simulink model "Simulation"  (R2018b)
settings: Solver=VariableStepAuto  StartTime=0.0  StopTime=tmax  RelTol=1e-3
values from neighbouring files (symbols this model uses):
  BPden = [1 alpha]    [RunSimulation.m]
  BPnum = [0.3 alpha]    [RunSimulation.m]
  c = 250    [RunSimulation.m]
  Fb = -1*m    (= -90000)    [RunSimulation.m]
  l = 18    [RunSimulation.m]
  m = 90000    [RunSimulation.m]    (also in TractionCurve.m = 22500)
  p0 = 0    [RunSimulation.m]
  Pres = 0/1000*[5.7/771 0 1.6]    [RunSimulation.m]
  RBD = 5    [RunSimulation.m]
  tl = .1    (= 0.1)    [RunSimulation.m]
  v0 = 100/3.6    (= 27.7777777778)    [RunSimulation.m]
  VBD = 3.5    [RunSimulation.m]
(part 2 of 3)

== system Simulation/Subsystem13/Wagon model2 ==
  p_BP : Inport
  Abs : Abs
  Constant : Constant  Value=m
  Divide : Product  Inputs=*/
  Gain : Gain  Gain=-1/(RBD-VBD)
  Gain1 : Gain  Gain=Fb
  Gravity : Gain  Gain=9.81
  Integrator : Integrator  InitialCondition=v0
  Product : Product
  Rate Limiter : RateLimiter  RisingSlewLimit=1/tf  FallingSlewLimit=-1/tl  SampleTimeMode=inherited
  Saturation : Saturate  UpperLimit=1  LowerLimit=0
  Strahl formula : Polyval  Coefs=Pres
  Sum1 : Sum  Inputs=|+-
  Transfer Fcn : TransferFcn  Numerator=BPnum  Denominator=BPden
  Transport Delay : TransportDelay  DelayTime=l/c  InitialOutput=p0
  Fres : Outport
  p_BP_out : Outport  Port=2
  wires:
  Sum1/1 -> Fres/1, Divide/1  "Fres"
  Strahl formula/1 -> Gravity/1
  Abs/1 -> Strahl formula/1
  Gravity/1 -> Product/2
  Product/1 -> Sum1/2  "Fw"
  Constant/1 -> Product/1, Divide/2
  Divide/1 -> Integrator/1  "a"
  p_BP/1 -> Gain/1, Transport Delay/1
  Gain/1 -> Saturation/1
  Gain1/1 -> Sum1/1
  Saturation/1 -> Rate Limiter/1
  Rate Limiter/1 -> Gain1/1
  Transport Delay/1 -> Transfer Fcn/1
  Transfer Fcn/1 -> p_BP_out/1
  Integrator/1 -> Abs/1  "v"

== system Simulation/Subsystem13/Wagon model3 ==
  p_BP : Inport
  Abs : Abs
  Constant : Constant  Value=m
  Divide : Product  Inputs=*/
  Gain : Gain  Gain=-1/(RBD-VBD)
  Gain1 : Gain  Gain=Fb
  Gravity : Gain  Gain=9.81
  Integrator : Integrator  InitialCondition=v0
  Product : Product
  Rate Limiter : RateLimiter  RisingSlewLimit=1/tf  FallingSlewLimit=-1/tl  SampleTimeMode=inherited
  Saturation : Saturate  UpperLimit=1  LowerLimit=0
  Strahl formula : Polyval  Coefs=Pres
  Sum1 : Sum  Inputs=|+-
  Transfer Fcn : TransferFcn  Numerator=BPnum  Denominator=BPden
  Transport Delay : TransportDelay  DelayTime=l/c  InitialOutput=p0
  Fres : Outport
  p_BP_out : Outport  Port=2
  wires:
  Sum1/1 -> Fres/1, Divide/1  "Fres"
  Strahl formula/1 -> Gravity/1
  Abs/1 -> Strahl formula/1
  Gravity/1 -> Product/2
  Product/1 -> Sum1/2  "Fw"
  Constant/1 -> Product/1, Divide/2
  Divide/1 -> Integrator/1  "a"
  p_BP/1 -> Gain/1, Transport Delay/1
  Gain/1 -> Saturation/1
  Gain1/1 -> Sum1/1
  Saturation/1 -> Rate Limiter/1
  Rate Limiter/1 -> Gain1/1
  Transport Delay/1 -> Transfer Fcn/1
  Transfer Fcn/1 -> p_BP_out/1
  Integrator/1 -> Abs/1  "v"

== system Simulation/Subsystem13/Wagon model4 ==
  p_BP : Inport
  Abs : Abs
  Constant : Constant  Value=m
  Divide : Product  Inputs=*/
  Gain : Gain  Gain=-1/(RBD-VBD)
  Gain1 : Gain  Gain=Fb
  Gravity : Gain  Gain=9.81
  Integrator : Integrator  InitialCondition=v0
  Product : Product
  Rate Limiter : RateLimiter  RisingSlewLimit=1/tf  FallingSlewLimit=-1/tl  SampleTimeMode=inherited
  Saturation : Saturate  UpperLimit=1  LowerLimit=0
  Strahl formula : Polyval  Coefs=Pres
  Sum1 : Sum  Inputs=|+-
  Transfer Fcn : TransferFcn  Numerator=BPnum  Denominator=BPden
  Transport Delay : TransportDelay  DelayTime=l/c  InitialOutput=p0
  Fres : Outport
  p_BP_out : Outport  Port=2
  wires:
  Sum1/1 -> Fres/1, Divide/1  "Fres"
  Strahl formula/1 -> Gravity/1
  Abs/1 -> Strahl formula/1
  Gravity/1 -> Product/2
  Product/1 -> Sum1/2  "Fw"
  Integrator/1 -> Abs/1  "v"
  Constant/1 -> Product/1, Divide/2
  Divide/1 -> Integrator/1  "a"
  p_BP/1 -> Gain/1, Transport Delay/1
  Gain/1 -> Saturation/1
  Gain1/1 -> Sum1/1
  Saturation/1 -> Rate Limiter/1
  Rate Limiter/1 -> Gain1/1
  Transfer Fcn/1 -> p_BP_out/1
  Transport Delay/1 -> Transfer Fcn/1

== system Simulation/Subsystem14/Wagon model ==
  p_BP : Inport
  Abs : Abs
  Constant : Constant  Value=m
  Divide : Product  Inputs=*/
  Gain : Gain  Gain=-1/(RBD-VBD)
  Gain1 : Gain  Gain=Fb
  Gravity : Gain  Gain=9.81
  Integrator : Integrator  InitialCondition=v0
  Product : Product
  Rate Limiter : RateLimiter  RisingSlewLimit=1/tf  FallingSlewLimit=-1/tl  SampleTimeMode=inherited
  Saturation : Saturate  UpperLimit=1  LowerLimit=0
  Strahl formula : Polyval  Coefs=Pres
  Sum1 : Sum  Inputs=|+-
  Transfer Fcn : TransferFcn  Numerator=BPnum  Denominator=BPden
  Transport Delay : TransportDelay  DelayTime=l/c  InitialOutput=p0
  Fres : Outport
  p_BP_out : Outport  Port=2
  wires:
  Sum1/1 -> Fres/1, Divide/1  "Fres"
  Strahl formula/1 -> Gravity/1
  Abs/1 -> Strahl formula/1
  Gravity/1 -> Product/2
  Product/1 -> Sum1/2  "Fw"
  Integrator/1 -> Abs/1  "v"
  Constant/1 -> Product/1, Divide/2
  Divide/1 -> Integrator/1  "a"
  p_BP/1 -> Gain/1, Transport Delay/1
  Gain/1 -> Saturation/1
  Gain1/1 -> Sum1/1
  Saturation/1 -> Rate Limiter/1
  Rate Limiter/1 -> Gain1/1
  Transfer Fcn/1 -> p_BP_out/1
  Transport Delay/1 -> Transfer Fcn/1

== system Simulation/Subsystem14/Wagon model1 ==
  p_BP : Inport
  Abs : Abs
  Constant : Constant  Value=m
  Divide : Product  Inputs=*/
  Gain : Gain  Gain=-1/(RBD-VBD)
  Gain1 : Gain  Gain=Fb
  Gravity : Gain  Gain=9.81
  Integrator : Integrator  InitialCondition=v0
  Product : Product
  Rate Limiter : RateLimiter  RisingSlewLimit=1/tf  FallingSlewLimit=-1/tl  SampleTimeMode=inherited
  Saturation : Saturate  UpperLimit=1  LowerLimit=0
  Strahl formula : Polyval  Coefs=Pres
  Sum1 : Sum  Inputs=|+-
  Transfer Fcn : TransferFcn  Numerator=BPnum  Denominator=BPden
  Transport Delay : TransportDelay  DelayTime=l/c  InitialOutput=p0
  Fres : Outport
  p_BP_out : Outport  Port=2
  wires:
  Sum1/1 -> Fres/1, Divide/1  "Fres"
  Strahl formula/1 -> Gravity/1
  Abs/1 -> Strahl formula/1
  Gravity/1 -> Product/2
  Product/1 -> Sum1/2  "Fw"
  Integrator/1 -> Abs/1  "v"
  Constant/1 -> Product/1, Divide/2
  Divide/1 -> Integrator/1  "a"
  p_BP/1 -> Gain/1, Transport Delay/1
  Gain/1 -> Saturation/1
  Gain1/1 -> Sum1/1
  Saturation/1 -> Rate Limiter/1
  Rate Limiter/1 -> Gain1/1
  Transport Delay/1 -> Transfer Fcn/1
  Transfer Fcn/1 -> p_BP_out/1

== system Simulation/Subsystem14/Wagon model2 ==
  p_BP : Inport
  Abs : Abs
  Constant : Constant  Value=m
  Divide : Product  Inputs=*/
  Gain : Gain  Gain=-1/(RBD-VBD)
  Gain1 : Gain  Gain=Fb
  Gravity : Gain  Gain=9.81
  Integrator : Integrator  InitialCondition=v0
  Product : Product
  Rate Limiter : RateLimiter  RisingSlewLimit=1/tf  FallingSlewLimit=-1/tl  SampleTimeMode=inherited
  Saturation : Saturate  UpperLimit=1  LowerLimit=0
  Strahl formula : Polyval  Coefs=Pres
  Sum1 : Sum  Inputs=|+-
  Transfer Fcn : TransferFcn  Numerator=BPnum  Denominator=BPden
  Transport Delay : TransportDelay  DelayTime=l/c  InitialOutput=p0
  Fres : Outport
  p_BP_out : Outport  Port=2
  wires:
  Sum1/1 -> Fres/1, Divide/1  "Fres"
  Strahl formula/1 -> Gravity/1
  Abs/1 -> Strahl formula/1
  Gravity/1 -> Product/2
  Product/1 -> Sum1/2  "Fw"
  Constant/1 -> Product/1, Divide/2
  Divide/1 -> Integrator/1  "a"
  p_BP/1 -> Gain/1, Transport Delay/1
  Gain/1 -> Saturation/1
  Gain1/1 -> Sum1/1
  Saturation/1 -> Rate Limiter/1
  Rate Limiter/1 -> Gain1/1
  Transport Delay/1 -> Transfer Fcn/1
  Transfer Fcn/1 -> p_BP_out/1
  Integrator/1 -> Abs/1  "v"

== system Simulation/Subsystem14/Wagon model3 ==
  p_BP : Inport
  Abs : Abs
  Constant : Constant  Value=m
  Divide : Product  Inputs=*/
  Gain : Gain  Gain=-1/(RBD-VBD)
  Gain1 : Gain  Gain=Fb
  Gravity : Gain  Gain=9.81
  Integrator : Integrator  InitialCondition=v0
  Product : Product
  Rate Limiter : RateLimiter  RisingSlewLimit=1/tf  FallingSlewLimit=-1/tl  SampleTimeMode=inherited
  Saturation : Saturate  UpperLimit=1  LowerLimit=0
  Strahl formula : Polyval  Coefs=Pres
  Sum1 : Sum  Inputs=|+-
  Transfer Fcn : TransferFcn  Numerator=BPnum  Denominator=BPden
  Transport Delay : TransportDelay  DelayTime=l/c  InitialOutput=p0
  Fres : Outport
  p_BP_out : Outport  Port=2
  wires:
  Sum1/1 -> Fres/1, Divide/1  "Fres"
  Strahl formula/1 -> Gravity/1
  Abs/1 -> Strahl formula/1
  Gravity/1 -> Product/2
  Product/1 -> Sum1/2  "Fw"
  Constant/1 -> Product/1, Divide/2
  Divide/1 -> Integrator/1  "a"
  p_BP/1 -> Gain/1, Transport Delay/1
  Gain/1 -> Saturation/1
  Gain1/1 -> Sum1/1
  Saturation/1 -> Rate Limiter/1
  Rate Limiter/1 -> Gain1/1
  Transport Delay/1 -> Transfer Fcn/1
  Transfer Fcn/1 -> p_BP_out/1
  Integrator/1 -> Abs/1  "v"

== system Simulation/Subsystem14/Wagon model4 ==
  p_BP : Inport
  Abs : Abs
  Constant : Constant  Value=m
  Divide : Product  Inputs=*/
  Gain : Gain  Gain=-1/(RBD-VBD)
  Gain1 : Gain  Gain=Fb
  Gravity : Gain  Gain=9.81
  Integrator : Integrator  InitialCondition=v0
  Product : Product
  Rate Limiter : RateLimiter  RisingSlewLimit=1/tf  FallingSlewLimit=-1/tl  SampleTimeMode=inherited
  Saturation : Saturate  UpperLimit=1  LowerLimit=0
  Strahl formula : Polyval  Coefs=Pres
  Sum1 : Sum  Inputs=|+-
  Transfer Fcn : TransferFcn  Numerator=BPnum  Denominator=BPden
  Transport Delay : TransportDelay  DelayTime=l/c  InitialOutput=p0
  Fres : Outport
  p_BP_out : Outport  Port=2
  wires:
  Sum1/1 -> Fres/1, Divide/1  "Fres"
  Strahl formula/1 -> Gravity/1
  Abs/1 -> Strahl formula/1
  Gravity/1 -> Product/2
  Product/1 -> Sum1/2  "Fw"
  Integrator/1 -> Abs/1  "v"
  Constant/1 -> Product/1, Divide/2
  Divide/1 -> Integrator/1  "a"
  p_BP/1 -> Gain/1, Transport Delay/1
  Gain/1 -> Saturation/1
  Gain1/1 -> Sum1/1
  Saturation/1 -> Rate Limiter/1
  Rate Limiter/1 -> Gain1/1
  Transfer Fcn/1 -> p_BP_out/1
  Transport Delay/1 -> Transfer Fcn/1

== system Simulation/Subsystem15/Wagon model ==
  p_BP : Inport
  Abs : Abs
  Constant : Constant  Value=m
  Divide : Product  Inputs=*/
  Gain : Gain  Gain=-1/(RBD-VBD)
  Gain1 : Gain  Gain=Fb
  Gravity : Gain  Gain=9.81
  Integrator : Integrator  InitialCondition=v0
  Product : Product
  Rate Limiter : RateLimiter  RisingSlewLimit=1/tf  FallingSlewLimit=-1/tl  SampleTimeMode=inherited
  Saturation : Saturate  UpperLimit=1  LowerLimit=0
  Strahl formula : Polyval  Coefs=Pres
  Sum1 : Sum  Inputs=|+-
  Transfer Fcn : TransferFcn  Numerator=BPnum  Denominator=BPden
  Transport Delay : TransportDelay  DelayTime=l/c  InitialOutput=p0
  Fres : Outport
  p_BP_out : Outport  Port=2
  wires:
  Sum1/1 -> Fres/1, Divide/1  "Fres"
  Strahl formula/1 -> Gravity/1
  Abs/1 -> Strahl formula/1
  Gravity/1 -> Product/2
  Product/1 -> Sum1/2  "Fw"
  Integrator/1 -> Abs/1  "v"
  Constant/1 -> Product/1, Divide/2
  Divide/1 -> Integrator/1  "a"
  p_BP/1 -> Gain/1, Transport Delay/1
  Gain/1 -> Saturation/1
  Gain1/1 -> Sum1/1
  Saturation/1 -> Rate Limiter/1
  Rate Limiter/1 -> Gain1/1
  Transfer Fcn/1 -> p_BP_out/1
  Transport Delay/1 -> Transfer Fcn/1

== system Simulation/Subsystem15/Wagon model1 ==
  p_BP : Inport
  Abs : Abs
  Constant : Constant  Value=m
  Divide : Product  Inputs=*/
  Gain : Gain  Gain=-1/(RBD-VBD)
  Gain1 : Gain  Gain=Fb
  Gravity : Gain  Gain=9.81
  Integrator : Integrator  InitialCondition=v0
  Product : Product
  Rate Limiter : RateLimiter  RisingSlewLimit=1/tf  FallingSlewLimit=-1/tl  SampleTimeMode=inherited
  Saturation : Saturate  UpperLimit=1  LowerLimit=0
  Strahl formula : Polyval  Coefs=Pres
  Sum1 : Sum  Inputs=|+-
  Transfer Fcn : TransferFcn  Numerator=BPnum  Denominator=BPden
  Transport Delay : TransportDelay  DelayTime=l/c  InitialOutput=p0
  Fres : Outport
  p_BP_out : Outport  Port=2
  wires:
  Sum1/1 -> Fres/1, Divide/1  "Fres"
  Strahl formula/1 -> Gravity/1
  Abs/1 -> Strahl formula/1
  Gravity/1 -> Product/2
  Product/1 -> Sum1/2  "Fw"
  Integrator/1 -> Abs/1  "v"
  Constant/1 -> Product/1, Divide/2
  Divide/1 -> Integrator/1  "a"
  p_BP/1 -> Gain/1, Transport Delay/1
  Gain/1 -> Saturation/1
  Gain1/1 -> Sum1/1
  Saturation/1 -> Rate Limiter/1
  Rate Limiter/1 -> Gain1/1
  Transport Delay/1 -> Transfer Fcn/1
  Transfer Fcn/1 -> p_BP_out/1

== system Simulation/Subsystem15/Wagon model2 ==
  p_BP : Inport
  Abs : Abs
  Constant : Constant  Value=m
  Divide : Product  Inputs=*/
  Gain : Gain  Gain=-1/(RBD-VBD)
  Gain1 : Gain  Gain=Fb
  Gravity : Gain  Gain=9.81
  Integrator : Integrator  InitialCondition=v0
  Product : Product
  Rate Limiter : RateLimiter  RisingSlewLimit=1/tf  FallingSlewLimit=-1/tl  SampleTimeMode=inherited
  Saturation : Saturate  UpperLimit=1  LowerLimit=0
  Strahl formula : Polyval  Coefs=Pres
  Sum1 : Sum  Inputs=|+-
  Transfer Fcn : TransferFcn  Numerator=BPnum  Denominator=BPden
  Transport Delay : TransportDelay  DelayTime=l/c  InitialOutput=p0
  Fres : Outport
  p_BP_out : Outport  Port=2
  wires:
  Sum1/1 -> Fres/1, Divide/1  "Fres"
  Strahl formula/1 -> Gravity/1
  Abs/1 -> Strahl formula/1
  Gravity/1 -> Product/2
  Product/1 -> Sum1/2  "Fw"
  Constant/1 -> Product/1, Divide/2
  Divide/1 -> Integrator/1  "a"
  p_BP/1 -> Gain/1, Transport Delay/1
  Gain/1 -> Saturation/1
  Gain1/1 -> Sum1/1
  Saturation/1 -> Rate Limiter/1
  Rate Limiter/1 -> Gain1/1
  Transport Delay/1 -> Transfer Fcn/1
  Transfer Fcn/1 -> p_BP_out/1
  Integrator/1 -> Abs/1  "v"

== system Simulation/Subsystem15/Wagon model3 ==
  p_BP : Inport
  Abs : Abs
  Constant : Constant  Value=m
  Divide : Product  Inputs=*/
  Gain : Gain  Gain=-1/(RBD-VBD)
  Gain1 : Gain  Gain=Fb
  Gravity : Gain  Gain=9.81
  Integrator : Integrator  InitialCondition=v0
  Product : Product
  Rate Limiter : RateLimiter  RisingSlewLimit=1/tf  FallingSlewLimit=-1/tl  SampleTimeMode=inherited
  Saturation : Saturate  UpperLimit=1  LowerLimit=0
  Strahl formula : Polyval  Coefs=Pres
  Sum1 : Sum  Inputs=|+-
  Transfer Fcn : TransferFcn  Numerator=BPnum  Denominator=BPden
  Transport Delay : TransportDelay  DelayTime=l/c  InitialOutput=p0
  Fres : Outport
  p_BP_out : Outport  Port=2
  wires:
  Sum1/1 -> Fres/1, Divide/1  "Fres"
  Strahl formula/1 -> Gravity/1
  Abs/1 -> Strahl formula/1
  Gravity/1 -> Product/2
  Product/1 -> Sum1/2  "Fw"
  Integrator/1 -> Abs/1  "v"
  Constant/1 -> Product/1, Divide/2
  Divide/1 -> Integrator/1  "a"
  p_BP/1 -> Gain/1, Transport Delay/1
  Gain/1 -> Saturation/1
  Gain1/1 -> Sum1/1
  Saturation/1 -> Rate Limiter/1
  Rate Limiter/1 -> Gain1/1
  Transport Delay/1 -> Transfer Fcn/1
  Transfer Fcn/1 -> p_BP_out/1

== system Simulation/Subsystem15/Wagon model4 ==
  p_BP : Inport
  Abs : Abs
  Constant : Constant  Value=m
  Divide : Product  Inputs=*/
  Gain : Gain  Gain=-1/(RBD-VBD)
  Gain1 : Gain  Gain=Fb
  Gravity : Gain  Gain=9.81
  Integrator : Integrator  InitialCondition=v0
  Product : Product
  Rate Limiter : RateLimiter  RisingSlewLimit=1/tf  FallingSlewLimit=-1/tl  SampleTimeMode=inherited
  Saturation : Saturate  UpperLimit=1  LowerLimit=0
  Strahl formula : Polyval  Coefs=Pres
  Sum1 : Sum  Inputs=|+-
  Transfer Fcn : TransferFcn  Numerator=BPnum  Denominator=BPden
  Transport Delay : TransportDelay  DelayTime=l/c  InitialOutput=p0
  Fres : Outport
  p_BP_out : Outport  Port=2
  wires:
  Sum1/1 -> Fres/1, Divide/1  "Fres"
  Strahl formula/1 -> Gravity/1
  Abs/1 -> Strahl formula/1
  Gravity/1 -> Product/2
  Product/1 -> Sum1/2  "Fw"
  Integrator/1 -> Abs/1  "v"
  Constant/1 -> Product/1, Divide/2
  Divide/1 -> Integrator/1  "a"
  p_BP/1 -> Gain/1, Transport Delay/1
  Gain/1 -> Saturation/1
  Gain1/1 -> Sum1/1
  Saturation/1 -> Rate Limiter/1
  Rate Limiter/1 -> Gain1/1
  Transfer Fcn/1 -> p_BP_out/1
  Transport Delay/1 -> Transfer Fcn/1

== system Simulation/Subsystem2/Wagon model ==
  p_BP : Inport
  Abs : Abs
  Constant : Constant  Value=m
  Divide : Product  Inputs=*/
  Gain : Gain  Gain=-1/(RBD-VBD)
  Gain1 : Gain  Gain=Fb
  Gravity : Gain  Gain=9.81
  Integrator : Integrator  InitialCondition=v0
  Product : Product
  Rate Limiter : RateLimiter  RisingSlewLimit=1/tf  FallingSlewLimit=-1/tl  SampleTimeMode=inherited
  Saturation : Saturate  UpperLimit=1  LowerLimit=0
  Strahl formula : Polyval  Coefs=Pres
  Sum1 : Sum  Inputs=|+-
  Transfer Fcn : TransferFcn  Numerator=BPnum  Denominator=BPden
  Transport Delay : TransportDelay  DelayTime=l/c  InitialOutput=p0
  Fres : Outport
  p_BP_out : Outport  Port=2
  wires:
  Sum1/1 -> Fres/1, Divide/1  "Fres"
  Strahl formula/1 -> Gravity/1
  Abs/1 -> Strahl formula/1
  Gravity/1 -> Product/2
  Product/1 -> Sum1/2  "Fw"
  Integrator/1 -> Abs/1  "v"
  Constant/1 -> Product/1, Divide/2
  Divide/1 -> Integrator/1  "a"
  p_BP/1 -> Gain/1, Transport Delay/1
  Gain/1 -> Saturation/1
  Gain1/1 -> Sum1/1
  Saturation/1 -> Rate Limiter/1
  Rate Limiter/1 -> Gain1/1
  Transfer Fcn/1 -> p_BP_out/1
  Transport Delay/1 -> Transfer Fcn/1

== system Simulation/Subsystem2/Wagon model1 ==
  p_BP : Inport
  Abs : Abs
  Constant : Constant  Value=m
  Divide : Product  Inputs=*/
  Gain : Gain  Gain=-1/(RBD-VBD)
  Gain1 : Gain  Gain=Fb
  Gravity : Gain  Gain=9.81
  Integrator : Integrator  InitialCondition=v0
  Product : Product
  Rate Limiter : RateLimiter  RisingSlewLimit=1/tf  FallingSlewLimit=-1/tl  SampleTimeMode=inherited
  Saturation : Saturate  UpperLimit=1  LowerLimit=0
  Strahl formula : Polyval  Coefs=Pres
  Sum1 : Sum  Inputs=|+-
  Transfer Fcn : TransferFcn  Numerator=BPnum  Denominator=BPden
  Transport Delay : TransportDelay  DelayTime=l/c  InitialOutput=p0
  Fres : Outport
  p_BP_out : Outport  Port=2
  wires:
  Sum1/1 -> Fres/1, Divide/1  "Fres"
  Strahl formula/1 -> Gravity/1
  Abs/1 -> Strahl formula/1
  Gravity/1 -> Product/2
  Product/1 -> Sum1/2  "Fw"
  Integrator/1 -> Abs/1  "v"
  Constant/1 -> Product/1, Divide/2
  Divide/1 -> Integrator/1  "a"
  p_BP/1 -> Gain/1, Transport Delay/1
  Gain/1 -> Saturation/1
  Gain1/1 -> Sum1/1
  Saturation/1 -> Rate Limiter/1
  Rate Limiter/1 -> Gain1/1
  Transport Delay/1 -> Transfer Fcn/1
  Transfer Fcn/1 -> p_BP_out/1

== system Simulation/Subsystem2/Wagon model2 ==
  p_BP : Inport
  Abs : Abs
  Constant : Constant  Value=m
  Divide : Product  Inputs=*/
  Gain : Gain  Gain=-1/(RBD-VBD)
  Gain1 : Gain  Gain=Fb
  Gravity : Gain  Gain=9.81
  Integrator : Integrator  InitialCondition=v0
  Product : Product
  Rate Limiter : RateLimiter  RisingSlewLimit=1/tf  FallingSlewLimit=-1/tl  SampleTimeMode=inherited
  Saturation : Saturate  UpperLimit=1  LowerLimit=0
  Strahl formula : Polyval  Coefs=Pres
  Sum1 : Sum  Inputs=|+-
  Transfer Fcn : TransferFcn  Numerator=BPnum  Denominator=BPden
  Transport Delay : TransportDelay  DelayTime=l/c  InitialOutput=p0
  Fres : Outport
  p_BP_out : Outport  Port=2
  wires:
  Sum1/1 -> Fres/1, Divide/1  "Fres"
  Strahl formula/1 -> Gravity/1
  Abs/1 -> Strahl formula/1
  Gravity/1 -> Product/2
  Product/1 -> Sum1/2  "Fw"
  Constant/1 -> Product/1, Divide/2
  Divide/1 -> Integrator/1  "a"
  p_BP/1 -> Gain/1, Transport Delay/1
  Gain/1 -> Saturation/1
  Gain1/1 -> Sum1/1
  Saturation/1 -> Rate Limiter/1
  Rate Limiter/1 -> Gain1/1
  Transport Delay/1 -> Transfer Fcn/1
  Transfer Fcn/1 -> p_BP_out/1
  Integrator/1 -> Abs/1  "v"

== system Simulation/Subsystem2/Wagon model3 ==
  p_BP : Inport
  Abs : Abs
  Constant : Constant  Value=m
  Divide : Product  Inputs=*/
  Gain : Gain  Gain=-1/(RBD-VBD)
  Gain1 : Gain  Gain=Fb
  Gravity : Gain  Gain=9.81
  Integrator : Integrator  InitialCondition=v0
  Product : Product
  Rate Limiter : RateLimiter  RisingSlewLimit=1/tf  FallingSlewLimit=-1/tl  SampleTimeMode=inherited
  Saturation : Saturate  UpperLimit=1  LowerLimit=0
  Strahl formula : Polyval  Coefs=Pres
  Sum1 : Sum  Inputs=|+-
  Transfer Fcn : TransferFcn  Numerator=BPnum  Denominator=BPden
  Transport Delay : TransportDelay  DelayTime=l/c  InitialOutput=p0
  Fres : Outport
  p_BP_out : Outport  Port=2
  wires:
  Sum1/1 -> Fres/1, Divide/1  "Fres"
  Strahl formula/1 -> Gravity/1
  Abs/1 -> Strahl formula/1
  Gravity/1 -> Product/2
  Product/1 -> Sum1/2  "Fw"
  Constant/1 -> Product/1, Divide/2
  Divide/1 -> Integrator/1  "a"
  p_BP/1 -> Gain/1, Transport Delay/1
  Gain/1 -> Saturation/1
  Gain1/1 -> Sum1/1
  Saturation/1 -> Rate Limiter/1
  Rate Limiter/1 -> Gain1/1
  Transport Delay/1 -> Transfer Fcn/1
  Transfer Fcn/1 -> p_BP_out/1
  Integrator/1 -> Abs/1  "v"

== system Simulation/Subsystem2/Wagon model4 ==
  p_BP : Inport
  Abs : Abs
  Constant : Constant  Value=m
  Divide : Product  Inputs=*/
  Gain : Gain  Gain=-1/(RBD-VBD)
  Gain1 : Gain  Gain=Fb
  Gravity : Gain  Gain=9.81
  Integrator : Integrator  InitialCondition=v0
  Product : Product
  Rate Limiter : RateLimiter  RisingSlewLimit=1/tf  FallingSlewLimit=-1/tl  SampleTimeMode=inherited
  Saturation : Saturate  UpperLimit=1  LowerLimit=0
  Strahl formula : Polyval  Coefs=Pres
  Sum1 : Sum  Inputs=|+-
  Transfer Fcn : TransferFcn  Numerator=BPnum  Denominator=BPden
  Transport Delay : TransportDelay  DelayTime=l/c  InitialOutput=p0
  Fres : Outport
  p_BP_out : Outport  Port=2
  wires:
  Sum1/1 -> Fres/1, Divide/1  "Fres"
  Strahl formula/1 -> Gravity/1
  Abs/1 -> Strahl formula/1
  Gravity/1 -> Product/2
  Product/1 -> Sum1/2  "Fw"
  Integrator/1 -> Abs/1  "v"
  Constant/1 -> Product/1, Divide/2
  Divide/1 -> Integrator/1  "a"
  p_BP/1 -> Gain/1, Transport Delay/1
  Gain/1 -> Saturation/1
  Gain1/1 -> Sum1/1
  Saturation/1 -> Rate Limiter/1
  Rate Limiter/1 -> Gain1/1
  Transfer Fcn/1 -> p_BP_out/1
  Transport Delay/1 -> Transfer Fcn/1

== system Simulation/Subsystem3/Wagon model ==
  p_BP : Inport
  Abs : Abs
  Constant : Constant  Value=m
  Divide : Product  Inputs=*/
  Gain : Gain  Gain=-1/(RBD-VBD)
  Gain1 : Gain  Gain=Fb
  Gravity : Gain  Gain=9.81
  Integrator : Integrator  InitialCondition=v0
  Product : Product
  Rate Limiter : RateLimiter  RisingSlewLimit=1/tf  FallingSlewLimit=-1/tl  SampleTimeMode=inherited
  Saturation : Saturate  UpperLimit=1  LowerLimit=0
  Strahl formula : Polyval  Coefs=Pres
  Sum1 : Sum  Inputs=|+-
  Transfer Fcn : TransferFcn  Numerator=BPnum  Denominator=BPden
  Transport Delay : TransportDelay  DelayTime=l/c  InitialOutput=p0
  Fres : Outport
  p_BP_out : Outport  Port=2
  wires:
  Sum1/1 -> Fres/1, Divide/1  "Fres"
  Strahl formula/1 -> Gravity/1
  Abs/1 -> Strahl formula/1
  Gravity/1 -> Product/2
  Product/1 -> Sum1/2  "Fw"
  Integrator/1 -> Abs/1  "v"
  Constant/1 -> Product/1, Divide/2
  Divide/1 -> Integrator/1  "a"
  p_BP/1 -> Gain/1, Transport Delay/1
  Gain/1 -> Saturation/1
  Gain1/1 -> Sum1/1
  Saturation/1 -> Rate Limiter/1
  Rate Limiter/1 -> Gain1/1
  Transfer Fcn/1 -> p_BP_out/1
  Transport Delay/1 -> Transfer Fcn/1

== system Simulation/Subsystem3/Wagon model1 ==
  p_BP : Inport
  Abs : Abs
  Constant : Constant  Value=m
  Divide : Product  Inputs=*/
  Gain : Gain  Gain=-1/(RBD-VBD)
  Gain1 : Gain  Gain=Fb
  Gravity : Gain  Gain=9.81
  Integrator : Integrator  InitialCondition=v0
  Product : Product
  Rate Limiter : RateLimiter  RisingSlewLimit=1/tf  FallingSlewLimit=-1/tl  SampleTimeMode=inherited
  Saturation : Saturate  UpperLimit=1  LowerLimit=0
  Strahl formula : Polyval  Coefs=Pres
  Sum1 : Sum  Inputs=|+-
  Transfer Fcn : TransferFcn  Numerator=BPnum  Denominator=BPden
  Transport Delay : TransportDelay  DelayTime=l/c  InitialOutput=p0
  Fres : Outport
  p_BP_out : Outport  Port=2
  wires:
  Sum1/1 -> Fres/1, Divide/1  "Fres"
  Strahl formula/1 -> Gravity/1
  Abs/1 -> Strahl formula/1
  Gravity/1 -> Product/2
  Product/1 -> Sum1/2  "Fw"
  Integrator/1 -> Abs/1  "v"
  Constant/1 -> Product/1, Divide/2
  Divide/1 -> Integrator/1  "a"
  p_BP/1 -> Gain/1, Transport Delay/1
  Gain/1 -> Saturation/1
  Gain1/1 -> Sum1/1
  Saturation/1 -> Rate Limiter/1
  Rate Limiter/1 -> Gain1/1
  Transport Delay/1 -> Transfer Fcn/1
  Transfer Fcn/1 -> p_BP_out/1

== system Simulation/Subsystem3/Wagon model2 ==
  p_BP : Inport
  Abs : Abs
  Constant : Constant  Value=m
  Divide : Product  Inputs=*/
  Gain : Gain  Gain=-1/(RBD-VBD)
  Gain1 : Gain  Gain=Fb
  Gravity : Gain  Gain=9.81
  Integrator : Integrator  InitialCondition=v0
  Product : Product
  Rate Limiter : RateLimiter  RisingSlewLimit=1/tf  FallingSlewLimit=-1/tl  SampleTimeMode=inherited
  Saturation : Saturate  UpperLimit=1  LowerLimit=0
  Strahl formula : Polyval  Coefs=Pres
  Sum1 : Sum  Inputs=|+-
  Transfer Fcn : TransferFcn  Numerator=BPnum  Denominator=BPden
  Transport Delay : TransportDelay  DelayTime=l/c  InitialOutput=p0
  Fres : Outport
  p_BP_out : Outport  Port=2
  wires:
  Sum1/1 -> Fres/1, Divide/1  "Fres"
  Strahl formula/1 -> Gravity/1
  Abs/1 -> Strahl formula/1
  Gravity/1 -> Product/2
  Product/1 -> Sum1/2  "Fw"
  Constant/1 -> Product/1, Divide/2
  Divide/1 -> Integrator/1  "a"
  p_BP/1 -> Gain/1, Transport Delay/1
  Gain/1 -> Saturation/1
  Gain1/1 -> Sum1/1
  Saturation/1 -> Rate Limiter/1
  Rate Limiter/1 -> Gain1/1
  Transport Delay/1 -> Transfer Fcn/1
  Transfer Fcn/1 -> p_BP_out/1
  Integrator/1 -> Abs/1  "v"

== system Simulation/Subsystem3/Wagon model3 ==
  p_BP : Inport
  Abs : Abs
  Constant : Constant  Value=m
  Divide : Product  Inputs=*/
  Gain : Gain  Gain=-1/(RBD-VBD)
  Gain1 : Gain  Gain=Fb
  Gravity : Gain  Gain=9.81
  Integrator : Integrator  InitialCondition=v0
  Product : Product
  Rate Limiter : RateLimiter  RisingSlewLimit=1/tf  FallingSlewLimit=-1/tl  SampleTimeMode=inherited
  Saturation : Saturate  UpperLimit=1  LowerLimit=0
  Strahl formula : Polyval  Coefs=Pres
  Sum1 : Sum  Inputs=|+-
  Transfer Fcn : TransferFcn  Numerator=BPnum  Denominator=BPden
  Transport Delay : TransportDelay  DelayTime=l/c  InitialOutput=p0
  Fres : Outport
  p_BP_out : Outport  Port=2
  wires:
  Sum1/1 -> Fres/1, Divide/1  "Fres"
  Strahl formula/1 -> Gravity/1
  Abs/1 -> Strahl formula/1
  Gravity/1 -> Product/2
  Product/1 -> Sum1/2  "Fw"
  Constant/1 -> Product/1, Divide/2
  Divide/1 -> Integrator/1  "a"
  p_BP/1 -> Gain/1, Transport Delay/1
  Gain/1 -> Saturation/1
  Gain1/1 -> Sum1/1
  Saturation/1 -> Rate Limiter/1
  Rate Limiter/1 -> Gain1/1
  Transport Delay/1 -> Transfer Fcn/1
  Transfer Fcn/1 -> p_BP_out/1
  Integrator/1 -> Abs/1  "v"

== system Simulation/Subsystem3/Wagon model4 ==
  p_BP : Inport
  Abs : Abs
  Constant : Constant  Value=m
  Divide : Product  Inputs=*/
  Gain : Gain  Gain=-1/(RBD-VBD)
  Gain1 : Gain  Gain=Fb
  Gravity : Gain  Gain=9.81
  Integrator : Integrator  InitialCondition=v0
  Product : Product
  Rate Limiter : RateLimiter  RisingSlewLimit=1/tf  FallingSlewLimit=-1/tl  SampleTimeMode=inherited
  Saturation : Saturate  UpperLimit=1  LowerLimit=0
  Strahl formula : Polyval  Coefs=Pres
  Sum1 : Sum  Inputs=|+-
  Transfer Fcn : TransferFcn  Numerator=BPnum  Denominator=BPden
  Transport Delay : TransportDelay  DelayTime=l/c  InitialOutput=p0
  Fres : Outport
  p_BP_out : Outport  Port=2
  wires:
  Sum1/1 -> Fres/1, Divide/1  "Fres"
  Strahl formula/1 -> Gravity/1
  Abs/1 -> Strahl formula/1
  Gravity/1 -> Product/2
  Product/1 -> Sum1/2  "Fw"
  Integrator/1 -> Abs/1  "v"
  Constant/1 -> Product/1, Divide/2
  Divide/1 -> Integrator/1  "a"
  p_BP/1 -> Gain/1, Transport Delay/1
  Gain/1 -> Saturation/1
  Gain1/1 -> Sum1/1
  Saturation/1 -> Rate Limiter/1
  Rate Limiter/1 -> Gain1/1
  Transfer Fcn/1 -> p_BP_out/1
  Transport Delay/1 -> Transfer Fcn/1

== system Simulation/Subsystem4/Wagon model ==
  p_BP : Inport
  Abs : Abs
  Constant : Constant  Value=m
  Divide : Product  Inputs=*/
  Gain : Gain  Gain=-1/(RBD-VBD)
  Gain1 : Gain  Gain=Fb
  Gravity : Gain  Gain=9.81
  Integrator : Integrator  InitialCondition=v0
  Product : Product
  Rate Limiter : RateLimiter  RisingSlewLimit=1/tf  FallingSlewLimit=-1/tl  SampleTimeMode=inherited
  Saturation : Saturate  UpperLimit=1  LowerLimit=0
  Strahl formula : Polyval  Coefs=Pres
  Sum1 : Sum  Inputs=|+-
  Transfer Fcn : TransferFcn  Numerator=BPnum  Denominator=BPden
  Transport Delay : TransportDelay  DelayTime=l/c  InitialOutput=p0
  Fres : Outport
  p_BP_out : Outport  Port=2
  wires:
  Sum1/1 -> Fres/1, Divide/1  "Fres"
  Strahl formula/1 -> Gravity/1
  Abs/1 -> Strahl formula/1
  Gravity/1 -> Product/2
  Product/1 -> Sum1/2  "Fw"
  Integrator/1 -> Abs/1  "v"
  Constant/1 -> Product/1, Divide/2
  Divide/1 -> Integrator/1  "a"
  p_BP/1 -> Gain/1, Transport Delay/1
  Gain/1 -> Saturation/1
  Gain1/1 -> Sum1/1
  Saturation/1 -> Rate Limiter/1
  Rate Limiter/1 -> Gain1/1
  Transfer Fcn/1 -> p_BP_out/1
  Transport Delay/1 -> Transfer Fcn/1

== system Simulation/Subsystem4/Wagon model1 ==
  p_BP : Inport
  Abs : Abs
  Constant : Constant  Value=m
  Divide : Product  Inputs=*/
  Gain : Gain  Gain=-1/(RBD-VBD)
  Gain1 : Gain  Gain=Fb
  Gravity : Gain  Gain=9.81
  Integrator : Integrator  InitialCondition=v0
  Product : Product
  Rate Limiter : RateLimiter  RisingSlewLimit=1/tf  FallingSlewLimit=-1/tl  SampleTimeMode=inherited
  Saturation : Saturate  UpperLimit=1  LowerLimit=0
  Strahl formula : Polyval  Coefs=Pres
  Sum1 : Sum  Inputs=|+-
  Transfer Fcn : TransferFcn  Numerator=BPnum  Denominator=BPden
  Transport Delay : TransportDelay  DelayTime=l/c  InitialOutput=p0
  Fres : Outport
  p_BP_out : Outport  Port=2
  wires:
  Sum1/1 -> Fres/1, Divide/1  "Fres"
  Strahl formula/1 -> Gravity/1
  Abs/1 -> Strahl formula/1
  Gravity/1 -> Product/2
  Product/1 -> Sum1/2  "Fw"
  Integrator/1 -> Abs/1  "v"
  Constant/1 -> Product/1, Divide/2
  Divide/1 -> Integrator/1  "a"
  p_BP/1 -> Gain/1, Transport Delay/1
  Gain/1 -> Saturation/1
  Gain1/1 -> Sum1/1
  Saturation/1 -> Rate Limiter/1
  Rate Limiter/1 -> Gain1/1
  Transport Delay/1 -> Transfer Fcn/1
  Transfer Fcn/1 -> p_BP_out/1

== system Simulation/Subsystem4/Wagon model2 ==
  p_BP : Inport
  Abs : Abs
  Constant : Constant  Value=m
  Divide : Product  Inputs=*/
  Gain : Gain  Gain=-1/(RBD-VBD)
  Gain1 : Gain  Gain=Fb
  Gravity : Gain  Gain=9.81
  Integrator : Integrator  InitialCondition=v0
  Product : Product
  Rate Limiter : RateLimiter  RisingSlewLimit=1/tf  FallingSlewLimit=-1/tl  SampleTimeMode=inherited
  Saturation : Saturate  UpperLimit=1  LowerLimit=0
  Strahl formula : Polyval  Coefs=Pres
  Sum1 : Sum  Inputs=|+-
  Transfer Fcn : TransferFcn  Numerator=BPnum  Denominator=BPden
  Transport Delay : TransportDelay  DelayTime=l/c  InitialOutput=p0
  Fres : Outport
  p_BP_out : Outport  Port=2
  wires:
  Sum1/1 -> Fres/1, Divide/1  "Fres"
  Strahl formula/1 -> Gravity/1
  Abs/1 -> Strahl formula/1
  Gravity/1 -> Product/2
  Product/1 -> Sum1/2  "Fw"
  Constant/1 -> Product/1, Divide/2
  Divide/1 -> Integrator/1  "a"
  p_BP/1 -> Gain/1, Transport Delay/1
  Gain/1 -> Saturation/1
  Gain1/1 -> Sum1/1
  Saturation/1 -> Rate Limiter/1
  Rate Limiter/1 -> Gain1/1
  Transport Delay/1 -> Transfer Fcn/1
  Transfer Fcn/1 -> p_BP_out/1
  Integrator/1 -> Abs/1  "v"

== system Simulation/Subsystem4/Wagon model3 ==
  p_BP : Inport
  Abs : Abs
  Constant : Constant  Value=m
  Divide : Product  Inputs=*/
  Gain : Gain  Gain=-1/(RBD-VBD)
  Gain1 : Gain  Gain=Fb
  Gravity : Gain  Gain=9.81
  Integrator : Integrator  InitialCondition=v0
  Product : Product
  Rate Limiter : RateLimiter  RisingSlewLimit=1/tf  FallingSlewLimit=-1/tl  SampleTimeMode=inherited
  Saturation : Saturate  UpperLimit=1  LowerLimit=0
  Strahl formula : Polyval  Coefs=Pres
  Sum1 : Sum  Inputs=|+-
  Transfer Fcn : TransferFcn  Numerator=BPnum  Denominator=BPden
  Transport Delay : TransportDelay  DelayTime=l/c  InitialOutput=p0
  Fres : Outport
  p_BP_out : Outport  Port=2
  wires:
  Sum1/1 -> Fres/1, Divide/1  "Fres"
  Strahl formula/1 -> Gravity/1
  Abs/1 -> Strahl formula/1
  Gravity/1 -> Product/2
  Product/1 -> Sum1/2  "Fw"
  Constant/1 -> Product/1, Divide/2
  Divide/1 -> Integrator/1  "a"
  p_BP/1 -> Gain/1, Transport Delay/1
  Gain/1 -> Saturation/1
  Gain1/1 -> Sum1/1
  Saturation/1 -> Rate Limiter/1
  Rate Limiter/1 -> Gain1/1
  Transport Delay/1 -> Transfer Fcn/1
  Transfer Fcn/1 -> p_BP_out/1
  Integrator/1 -> Abs/1  "v"

== system Simulation/Subsystem4/Wagon model4 ==
  p_BP : Inport
  Abs : Abs
  Constant : Constant  Value=m
  Divide : Product  Inputs=*/
  Gain : Gain  Gain=-1/(RBD-VBD)
  Gain1 : Gain  Gain=Fb
  Gravity : Gain  Gain=9.81
  Integrator : Integrator  InitialCondition=v0
  Product : Product
  Rate Limiter : RateLimiter  RisingSlewLimit=1/tf  FallingSlewLimit=-1/tl  SampleTimeMode=inherited
  Saturation : Saturate  UpperLimit=1  LowerLimit=0
  Strahl formula : Polyval  Coefs=Pres
  Sum1 : Sum  Inputs=|+-
  Transfer Fcn : TransferFcn  Numerator=BPnum  Denominator=BPden
  Transport Delay : TransportDelay  DelayTime=l/c  InitialOutput=p0
  Fres : Outport
  p_BP_out : Outport  Port=2
  wires:
  Sum1/1 -> Fres/1, Divide/1  "Fres"
  Strahl formula/1 -> Gravity/1
  Abs/1 -> Strahl formula/1
  Gravity/1 -> Product/2
  Product/1 -> Sum1/2  "Fw"
  Integrator/1 -> Abs/1  "v"
  Constant/1 -> Product/1, Divide/2
  Divide/1 -> Integrator/1  "a"
  p_BP/1 -> Gain/1, Transport Delay/1
  Gain/1 -> Saturation/1
  Gain1/1 -> Sum1/1
  Saturation/1 -> Rate Limiter/1
  Rate Limiter/1 -> Gain1/1
  Transfer Fcn/1 -> p_BP_out/1
  Transport Delay/1 -> Transfer Fcn/1

== system Simulation/Subsystem5/Wagon model ==
  p_BP : Inport
  Abs : Abs
  Constant : Constant  Value=m
  Divide : Product  Inputs=*/
  Gain : Gain  Gain=-1/(RBD-VBD)
  Gain1 : Gain  Gain=Fb
  Gravity : Gain  Gain=9.81
  Integrator : Integrator  InitialCondition=v0
  Product : Product
  Rate Limiter : RateLimiter  RisingSlewLimit=1/tf  FallingSlewLimit=-1/tl  SampleTimeMode=inherited
  Saturation : Saturate  UpperLimit=1  LowerLimit=0
  Strahl formula : Polyval  Coefs=Pres
  Sum1 : Sum  Inputs=|+-
  Transfer Fcn : TransferFcn  Numerator=BPnum  Denominator=BPden
  Transport Delay : TransportDelay  DelayTime=l/c  InitialOutput=p0
  Fres : Outport
  p_BP_out : Outport  Port=2
  wires:
  Sum1/1 -> Fres/1, Divide/1  "Fres"
  Strahl formula/1 -> Gravity/1
  Abs/1 -> Strahl formula/1
  Gravity/1 -> Product/2
  Product/1 -> Sum1/2  "Fw"
  Integrator/1 -> Abs/1  "v"
  Constant/1 -> Product/1, Divide/2
  Divide/1 -> Integrator/1  "a"
  p_BP/1 -> Gain/1, Transport Delay/1
  Gain/1 -> Saturation/1
  Gain1/1 -> Sum1/1
  Saturation/1 -> Rate Limiter/1
  Rate Limiter/1 -> Gain1/1
  Transfer Fcn/1 -> p_BP_out/1
  Transport Delay/1 -> Transfer Fcn/1

== system Simulation/Subsystem5/Wagon model1 ==
  p_BP : Inport
  Abs : Abs
  Constant : Constant  Value=m
  Divide : Product  Inputs=*/
  Gain : Gain  Gain=-1/(RBD-VBD)
  Gain1 : Gain  Gain=Fb
  Gravity : Gain  Gain=9.81
  Integrator : Integrator  InitialCondition=v0
  Product : Product
  Rate Limiter : RateLimiter  RisingSlewLimit=1/tf  FallingSlewLimit=-1/tl  SampleTimeMode=inherited
  Saturation : Saturate  UpperLimit=1  LowerLimit=0
  Strahl formula : Polyval  Coefs=Pres
  Sum1 : Sum  Inputs=|+-
  Transfer Fcn : TransferFcn  Numerator=BPnum  Denominator=BPden
  Transport Delay : TransportDelay  DelayTime=l/c  InitialOutput=p0
  Fres : Outport
  p_BP_out : Outport  Port=2
  wires:
  Sum1/1 -> Fres/1, Divide/1  "Fres"
  Strahl formula/1 -> Gravity/1
  Abs/1 -> Strahl formula/1
  Gravity/1 -> Product/2
  Product/1 -> Sum1/2  "Fw"
  Integrator/1 -> Abs/1  "v"
  Constant/1 -> Product/1, Divide/2
  Divide/1 -> Integrator/1  "a"
  p_BP/1 -> Gain/1, Transport Delay/1
  Gain/1 -> Saturation/1
  Gain1/1 -> Sum1/1
  Saturation/1 -> Rate Limiter/1
  Rate Limiter/1 -> Gain1/1
  Transport Delay/1 -> Transfer Fcn/1
  Transfer Fcn/1 -> p_BP_out/1

== system Simulation/Subsystem5/Wagon model2 ==
  p_BP : Inport
  Abs : Abs
  Constant : Constant  Value=m
  Divide : Product  Inputs=*/
  Gain : Gain  Gain=-1/(RBD-VBD)
  Gain1 : Gain  Gain=Fb
  Gravity : Gain  Gain=9.81
  Integrator : Integrator  InitialCondition=v0
  Product : Product
  Rate Limiter : RateLimiter  RisingSlewLimit=1/tf  FallingSlewLimit=-1/tl  SampleTimeMode=inherited
  Saturation : Saturate  UpperLimit=1  LowerLimit=0
  Strahl formula : Polyval  Coefs=Pres
  Sum1 : Sum  Inputs=|+-
  Transfer Fcn : TransferFcn  Numerator=BPnum  Denominator=BPden
  Transport Delay : TransportDelay  DelayTime=l/c  InitialOutput=p0
  Fres : Outport
  p_BP_out : Outport  Port=2
  wires:
  Sum1/1 -> Fres/1, Divide/1  "Fres"
  Strahl formula/1 -> Gravity/1
  Abs/1 -> Strahl formula/1
  Gravity/1 -> Product/2
  Product/1 -> Sum1/2  "Fw"
  Constant/1 -> Product/1, Divide/2
  Divide/1 -> Integrator/1  "a"
  p_BP/1 -> Gain/1, Transport Delay/1
  Gain/1 -> Saturation/1
  Gain1/1 -> Sum1/1
  Saturation/1 -> Rate Limiter/1
  Rate Limiter/1 -> Gain1/1
  Transport Delay/1 -> Transfer Fcn/1
  Transfer Fcn/1 -> p_BP_out/1
  Integrator/1 -> Abs/1  "v"

== system Simulation/Subsystem5/Wagon model3 ==
  p_BP : Inport
  Abs : Abs
  Constant : Constant  Value=m
  Divide : Product  Inputs=*/
  Gain : Gain  Gain=-1/(RBD-VBD)
  Gain1 : Gain  Gain=Fb
  Gravity : Gain  Gain=9.81
  Integrator : Integrator  InitialCondition=v0
  Product : Product
  Rate Limiter : RateLimiter  RisingSlewLimit=1/tf  FallingSlewLimit=-1/tl  SampleTimeMode=inherited
  Saturation : Saturate  UpperLimit=1  LowerLimit=0
  Strahl formula : Polyval  Coefs=Pres
  Sum1 : Sum  Inputs=|+-
  Transfer Fcn : TransferFcn  Numerator=BPnum  Denominator=BPden
  Transport Delay : TransportDelay  DelayTime=l/c  InitialOutput=p0
  Fres : Outport
  p_BP_out : Outport  Port=2
  wires:
  Sum1/1 -> Fres/1, Divide/1  "Fres"
  Strahl formula/1 -> Gravity/1
  Abs/1 -> Strahl formula/1
  Gravity/1 -> Product/2
  Product/1 -> Sum1/2  "Fw"
  Constant/1 -> Product/1, Divide/2
  Divide/1 -> Integrator/1  "a"
  p_BP/1 -> Gain/1, Transport Delay/1
  Gain/1 -> Saturation/1
  Gain1/1 -> Sum1/1
  Saturation/1 -> Rate Limiter/1
  Rate Limiter/1 -> Gain1/1
  Transport Delay/1 -> Transfer Fcn/1
  Transfer Fcn/1 -> p_BP_out/1
  Integrator/1 -> Abs/1  "v"

== system Simulation/Subsystem5/Wagon model4 ==
  p_BP : Inport
  Abs : Abs
  Constant : Constant  Value=m
  Divide : Product  Inputs=*/
  Gain : Gain  Gain=-1/(RBD-VBD)
  Gain1 : Gain  Gain=Fb
  Gravity : Gain  Gain=9.81
  Integrator : Integrator  InitialCondition=v0
  Product : Product
  Rate Limiter : RateLimiter  RisingSlewLimit=1/tf  FallingSlewLimit=-1/tl  SampleTimeMode=inherited
  Saturation : Saturate  UpperLimit=1  LowerLimit=0
  Strahl formula : Polyval  Coefs=Pres
  Sum1 : Sum  Inputs=|+-
  Transfer Fcn : TransferFcn  Numerator=BPnum  Denominator=BPden
  Transport Delay : TransportDelay  DelayTime=l/c  InitialOutput=p0
  Fres : Outport
  p_BP_out : Outport  Port=2
  wires:
  Sum1/1 -> Fres/1, Divide/1  "Fres"
  Strahl formula/1 -> Gravity/1
  Abs/1 -> Strahl formula/1
  Gravity/1 -> Product/2
  Product/1 -> Sum1/2  "Fw"
  Integrator/1 -> Abs/1  "v"
  Constant/1 -> Product/1, Divide/2
  Divide/1 -> Integrator/1  "a"
  p_BP/1 -> Gain/1, Transport Delay/1
  Gain/1 -> Saturation/1
  Gain1/1 -> Sum1/1
  Saturation/1 -> Rate Limiter/1
  Rate Limiter/1 -> Gain1/1
  Transfer Fcn/1 -> p_BP_out/1
  Transport Delay/1 -> Transfer Fcn/1

== system Simulation/Subsystem6/Wagon model ==
  p_BP : Inport
  Abs : Abs
  Constant : Constant  Value=m
  Divide : Product  Inputs=*/
  Gain : Gain  Gain=-1/(RBD-VBD)
  Gain1 : Gain  Gain=Fb
  Gravity : Gain  Gain=9.81
  Integrator : Integrator  InitialCondition=v0
  Product : Product
  Rate Limiter : RateLimiter  RisingSlewLimit=1/tf  FallingSlewLimit=-1/tl  SampleTimeMode=inherited
  Saturation : Saturate  UpperLimit=1  LowerLimit=0
  Strahl formula : Polyval  Coefs=Pres
  Sum1 : Sum  Inputs=|+-
  Transfer Fcn : TransferFcn  Numerator=BPnum  Denominator=BPden
  Transport Delay : TransportDelay  DelayTime=l/c  InitialOutput=p0
  Fres : Outport
  p_BP_out : Outport  Port=2
  wires:
  Sum1/1 -> Fres/1, Divide/1  "Fres"
  Strahl formula/1 -> Gravity/1
  Abs/1 -> Strahl formula/1
  Gravity/1 -> Product/2
  Product/1 -> Sum1/2  "Fw"
  Integrator/1 -> Abs/1  "v"
  Constant/1 -> Product/1, Divide/2
  Divide/1 -> Integrator/1  "a"
  p_BP/1 -> Gain/1, Transport Delay/1
  Gain/1 -> Saturation/1
  Gain1/1 -> Sum1/1
  Saturation/1 -> Rate Limiter/1
  Rate Limiter/1 -> Gain1/1
  Transfer Fcn/1 -> p_BP_out/1
  Transport Delay/1 -> Transfer Fcn/1

== system Simulation/Subsystem6/Wagon model1 ==
  p_BP : Inport
  Abs : Abs
  Constant : Constant  Value=m
  Divide : Product  Inputs=*/
  Gain : Gain  Gain=-1/(RBD-VBD)
  Gain1 : Gain  Gain=Fb
  Gravity : Gain  Gain=9.81
  Integrator : Integrator  InitialCondition=v0
  Product : Product
  Rate Limiter : RateLimiter  RisingSlewLimit=1/tf  FallingSlewLimit=-1/tl  SampleTimeMode=inherited
  Saturation : Saturate  UpperLimit=1  LowerLimit=0
  Strahl formula : Polyval  Coefs=Pres
  Sum1 : Sum  Inputs=|+-
  Transfer Fcn : TransferFcn  Numerator=BPnum  Denominator=BPden
  Transport Delay : TransportDelay  DelayTime=l/c  InitialOutput=p0
  Fres : Outport
  p_BP_out : Outport  Port=2
  wires:
  Sum1/1 -> Fres/1, Divide/1  "Fres"
  Strahl formula/1 -> Gravity/1
  Abs/1 -> Strahl formula/1
  Gravity/1 -> Product/2
  Product/1 -> Sum1/2  "Fw"
  Integrator/1 -> Abs/1  "v"
  Constant/1 -> Product/1, Divide/2
  Divide/1 -> Integrator/1  "a"
  p_BP/1 -> Gain/1, Transport Delay/1
  Gain/1 -> Saturation/1
  Gain1/1 -> Sum1/1
  Saturation/1 -> Rate Limiter/1
  Rate Limiter/1 -> Gain1/1
  Transport Delay/1 -> Transfer Fcn/1
  Transfer Fcn/1 -> p_BP_out/1

== system Simulation/Subsystem6/Wagon model2 ==
  p_BP : Inport
  Abs : Abs
  Constant : Constant  Value=m
  Divide : Product  Inputs=*/
  Gain : Gain  Gain=-1/(RBD-VBD)
  Gain1 : Gain  Gain=Fb
  Gravity : Gain  Gain=9.81
  Integrator : Integrator  InitialCondition=v0
  Product : Product
  Rate Limiter : RateLimiter  RisingSlewLimit=1/tf  FallingSlewLimit=-1/tl  SampleTimeMode=inherited
  Saturation : Saturate  UpperLimit=1  LowerLimit=0
  Strahl formula : Polyval  Coefs=Pres
  Sum1 : Sum  Inputs=|+-
  Transfer Fcn : TransferFcn  Numerator=BPnum  Denominator=BPden
  Transport Delay : TransportDelay  DelayTime=l/c  InitialOutput=p0
  Fres : Outport
  p_BP_out : Outport  Port=2
  wires:
  Sum1/1 -> Fres/1, Divide/1  "Fres"
  Strahl formula/1 -> Gravity/1
  Abs/1 -> Strahl formula/1
  Gravity/1 -> Product/2
  Product/1 -> Sum1/2  "Fw"
  Constant/1 -> Product/1, Divide/2
  Divide/1 -> Integrator/1  "a"
  p_BP/1 -> Gain/1, Transport Delay/1
  Gain/1 -> Saturation/1
  Gain1/1 -> Sum1/1
  Saturation/1 -> Rate Limiter/1
  Rate Limiter/1 -> Gain1/1
  Transport Delay/1 -> Transfer Fcn/1
  Transfer Fcn/1 -> p_BP_out/1
  Integrator/1 -> Abs/1  "v"

== system Simulation/Subsystem6/Wagon model3 ==
  p_BP : Inport
  Abs : Abs
  Constant : Constant  Value=m
  Divide : Product  Inputs=*/
  Gain : Gain  Gain=-1/(RBD-VBD)
  Gain1 : Gain  Gain=Fb
  Gravity : Gain  Gain=9.81
  Integrator : Integrator  InitialCondition=v0
  Product : Product
  Rate Limiter : RateLimiter  RisingSlewLimit=1/tf  FallingSlewLimit=-1/tl  SampleTimeMode=inherited
  Saturation : Saturate  UpperLimit=1  LowerLimit=0
  Strahl formula : Polyval  Coefs=Pres
  Sum1 : Sum  Inputs=|+-
  Transfer Fcn : TransferFcn  Numerator=BPnum  Denominator=BPden
  Transport Delay : TransportDelay  DelayTime=l/c  InitialOutput=p0
  Fres : Outport
  p_BP_out : Outport  Port=2
  wires:
  Sum1/1 -> Fres/1, Divide/1  "Fres"
  Strahl formula/1 -> Gravity/1
  Abs/1 -> Strahl formula/1
  Gravity/1 -> Product/2
  Product/1 -> Sum1/2  "Fw"
  Constant/1 -> Product/1, Divide/2
  Divide/1 -> Integrator/1  "a"
  p_BP/1 -> Gain/1, Transport Delay/1
  Gain/1 -> Saturation/1
  Gain1/1 -> Sum1/1
  Saturation/1 -> Rate Limiter/1
  Rate Limiter/1 -> Gain1/1
  Transport Delay/1 -> Transfer Fcn/1
  Transfer Fcn/1 -> p_BP_out/1
  Integrator/1 -> Abs/1  "v"

== system Simulation/Subsystem6/Wagon model4 ==
  p_BP : Inport
  Abs : Abs
  Constant : Constant  Value=m
  Divide : Product  Inputs=*/
  Gain : Gain  Gain=-1/(RBD-VBD)
  Gain1 : Gain  Gain=Fb
  Gravity : Gain  Gain=9.81
  Integrator : Integrator  InitialCondition=v0
  Product : Product
  Rate Limiter : RateLimiter  RisingSlewLimit=1/tf  FallingSlewLimit=-1/tl  SampleTimeMode=inherited
  Saturation : Saturate  UpperLimit=1  LowerLimit=0
  Strahl formula : Polyval  Coefs=Pres
  Sum1 : Sum  Inputs=|+-
  Transfer Fcn : TransferFcn  Numerator=BPnum  Denominator=BPden
  Transport Delay : TransportDelay  DelayTime=l/c  InitialOutput=p0
  Fres : Outport
  p_BP_out : Outport  Port=2
  wires:
  Sum1/1 -> Fres/1, Divide/1  "Fres"
  Strahl formula/1 -> Gravity/1
  Abs/1 -> Strahl formula/1
  Gravity/1 -> Product/2
  Product/1 -> Sum1/2  "Fw"
  Integrator/1 -> Abs/1  "v"
  Constant/1 -> Product/1, Divide/2
  Divide/1 -> Integrator/1  "a"
  p_BP/1 -> Gain/1, Transport Delay/1
  Gain/1 -> Saturation/1
  Gain1/1 -> Sum1/1
  Saturation/1 -> Rate Limiter/1
  Rate Limiter/1 -> Gain1/1
  Transfer Fcn/1 -> p_BP_out/1
  Transport Delay/1 -> Transfer Fcn/1

== system Simulation/Subsystem7/Wagon model ==
  p_BP : Inport
  Abs : Abs
  Constant : Constant  Value=m
  Divide : Product  Inputs=*/
  Gain : Gain  Gain=-1/(RBD-VBD)
  Gain1 : Gain  Gain=Fb
  Gravity : Gain  Gain=9.81
  Integrator : Integrator  InitialCondition=v0
  Product : Product
  Rate Limiter : RateLimiter  RisingSlewLimit=1/tf  FallingSlewLimit=-1/tl  SampleTimeMode=inherited
  Saturation : Saturate  UpperLimit=1  LowerLimit=0
  Strahl formula : Polyval  Coefs=Pres
  Sum1 : Sum  Inputs=|+-
  Transfer Fcn : TransferFcn  Numerator=BPnum  Denominator=BPden
  Transport Delay : TransportDelay  DelayTime=l/c  InitialOutput=p0
  Fres : Outport
  p_BP_out : Outport  Port=2
  wires:
  Sum1/1 -> Fres/1, Divide/1  "Fres"
  Strahl formula/1 -> Gravity/1
  Abs/1 -> Strahl formula/1
  Gravity/1 -> Product/2
  Product/1 -> Sum1/2  "Fw"
  Integrator/1 -> Abs/1  "v"
  Constant/1 -> Product/1, Divide/2
  Divide/1 -> Integrator/1  "a"
  p_BP/1 -> Gain/1, Transport Delay/1
  Gain/1 -> Saturation/1
  Gain1/1 -> Sum1/1
  Saturation/1 -> Rate Limiter/1
  Rate Limiter/1 -> Gain1/1
  Transfer Fcn/1 -> p_BP_out/1
  Transport Delay/1 -> Transfer Fcn/1

== system Simulation/Subsystem7/Wagon model1 ==
  p_BP : Inport
  Abs : Abs
  Constant : Constant  Value=m
  Divide : Product  Inputs=*/
  Gain : Gain  Gain=-1/(RBD-VBD)
  Gain1 : Gain  Gain=Fb
  Gravity : Gain  Gain=9.81
  Integrator : Integrator  InitialCondition=v0
  Product : Product
  Rate Limiter : RateLimiter  RisingSlewLimit=1/tf  FallingSlewLimit=-1/tl  SampleTimeMode=inherited
  Saturation : Saturate  UpperLimit=1  LowerLimit=0
  Strahl formula : Polyval  Coefs=Pres
  Sum1 : Sum  Inputs=|+-
  Transfer Fcn : TransferFcn  Numerator=BPnum  Denominator=BPden
  Transport Delay : TransportDelay  DelayTime=l/c  InitialOutput=p0
  Fres : Outport
  p_BP_out : Outport  Port=2
  wires:
  Sum1/1 -> Fres/1, Divide/1  "Fres"
  Strahl formula/1 -> Gravity/1
  Abs/1 -> Strahl formula/1
  Gravity/1 -> Product/2
  Product/1 -> Sum1/2  "Fw"
  Integrator/1 -> Abs/1  "v"
  Constant/1 -> Product/1, Divide/2
  Divide/1 -> Integrator/1  "a"
  p_BP/1 -> Gain/1, Transport Delay/1
  Gain/1 -> Saturation/1
  Gain1/1 -> Sum1/1
  Saturation/1 -> Rate Limiter/1
  Rate Limiter/1 -> Gain1/1
  Transport Delay/1 -> Transfer Fcn/1
  Transfer Fcn/1 -> p_BP_out/1

== system Simulation/Subsystem7/Wagon model2 ==
  p_BP : Inport
  Abs : Abs
  Constant : Constant  Value=m
  Divide : Product  Inputs=*/
  Gain : Gain  Gain=-1/(RBD-VBD)
  Gain1 : Gain  Gain=Fb
  Gravity : Gain  Gain=9.81
  Integrator : Integrator  InitialCondition=v0
  Product : Product
  Rate Limiter : RateLimiter  RisingSlewLimit=1/tf  FallingSlewLimit=-1/tl  SampleTimeMode=inherited
  Saturation : Saturate  UpperLimit=1  LowerLimit=0
  Strahl formula : Polyval  Coefs=Pres
  Sum1 : Sum  Inputs=|+-
  Transfer Fcn : TransferFcn  Numerator=BPnum  Denominator=BPden
  Transport Delay : TransportDelay  DelayTime=l/c  InitialOutput=p0
  Fres : Outport
  p_BP_out : Outport  Port=2
  wires:
  Sum1/1 -> Fres/1, Divide/1  "Fres"
  Strahl formula/1 -> Gravity/1
  Abs/1 -> Strahl formula/1
  Gravity/1 -> Product/2
  Product/1 -> Sum1/2  "Fw"
  Constant/1 -> Product/1, Divide/2
  Divide/1 -> Integrator/1  "a"
  p_BP/1 -> Gain/1, Transport Delay/1
  Gain/1 -> Saturation/1
  Gain1/1 -> Sum1/1
  Saturation/1 -> Rate Limiter/1
  Rate Limiter/1 -> Gain1/1
  Transport Delay/1 -> Transfer Fcn/1
  Transfer Fcn/1 -> p_BP_out/1
  Integrator/1 -> Abs/1  "v"

== system Simulation/Subsystem7/Wagon model3 ==
  p_BP : Inport
  Abs : Abs
  Constant : Constant  Value=m
  Divide : Product  Inputs=*/
  Gain : Gain  Gain=-1/(RBD-VBD)
  Gain1 : Gain  Gain=Fb
  Gravity : Gain  Gain=9.81
  Integrator : Integrator  InitialCondition=v0
  Product : Product
  Rate Limiter : RateLimiter  RisingSlewLimit=1/tf  FallingSlewLimit=-1/tl  SampleTimeMode=inherited
  Saturation : Saturate  UpperLimit=1  LowerLimit=0
  Strahl formula : Polyval  Coefs=Pres
  Sum1 : Sum  Inputs=|+-
  Transfer Fcn : TransferFcn  Numerator=BPnum  Denominator=BPden
  Transport Delay : TransportDelay  DelayTime=l/c  InitialOutput=p0
  Fres : Outport
  p_BP_out : Outport  Port=2
  wires:
  Sum1/1 -> Fres/1, Divide/1  "Fres"
  Strahl formula/1 -> Gravity/1
  Abs/1 -> Strahl formula/1
  Gravity/1 -> Product/2
  Product/1 -> Sum1/2  "Fw"
  Integrator/1 -> Abs/1  "v"
  Constant/1 -> Product/1, Divide/2
  Divide/1 -> Integrator/1  "a"
  p_BP/1 -> Gain/1, Transport Delay/1
  Gain/1 -> Saturation/1
  Gain1/1 -> Sum1/1
  Saturation/1 -> Rate Limiter/1
  Rate Limiter/1 -> Gain1/1
  Transport Delay/1 -> Transfer Fcn/1
  Transfer Fcn/1 -> p_BP_out/1
